simulink model "wetCondition scenario 3"  (R2025a)
settings: Solver=VariableStepAuto  StartTime=0.0  StopTime=10.0  RelTol=1e-3
libraries: SignalEditorBlockLib x5
settings Model: Creator=josik  LastModifiedBy=josik

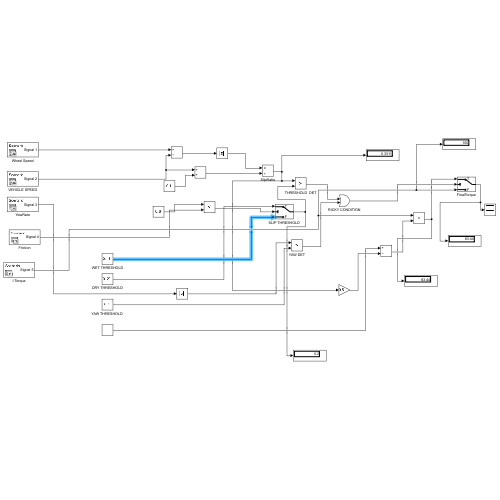
[thumbnail: Simulink's stored preview of the top-level diagram]
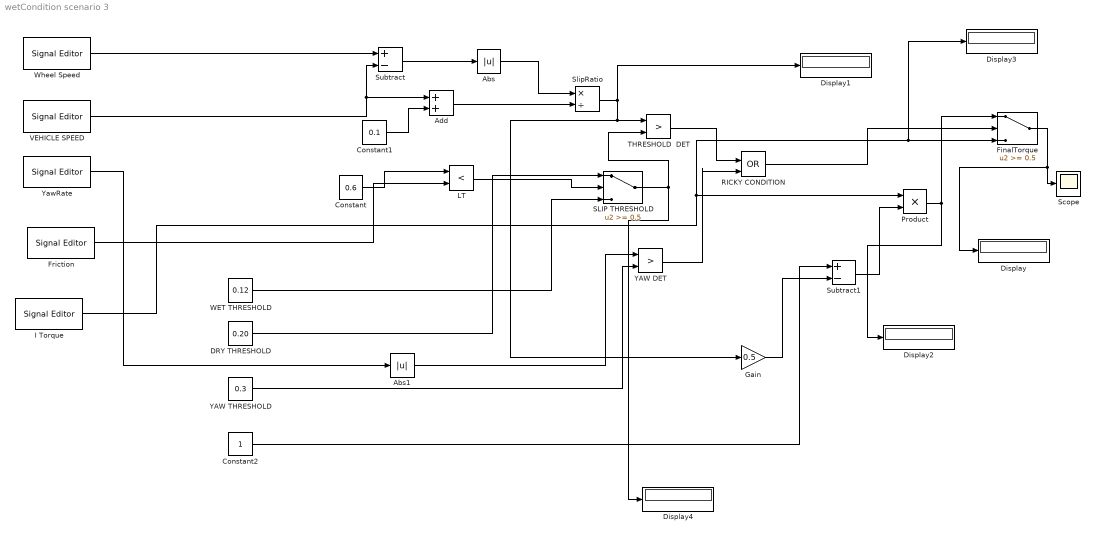
== system wetCondition scenario 3 ==
  Abs : Abs  SaturateOnIntegerOverflow=off
  Abs1 : Abs  SaturateOnIntegerOverflow=off
  Add : Sum
  Constant : Constant  Value=0.6
  Constant1 : Constant  Value=0.1
  Constant2 : Constant
  DRY THRESHOLD : Constant  Value=0.20
  Display{,1..4} (5 alike) : Display
  FinalTorque : Switch  Threshold=0.5  SaturateOnIntegerOverflow=off  InputSameDT=off
  Friction : SignalEditorBlockLib/Signal Editor  FileName=signal 4 sc 1.mat  ActiveScenario=Scenario  ActiveSignal=Signal 4  IsBus=off  OutputBusObjectStr=Bus: BusObject  SampleTime=0  ZeroCross=off  OutputAfterFinalValue=Setting to zero  Unit=inherit  PreserveSignalName=on  ApplySigPropsToAllScenarios=on  ApplySigPropsToAllSignals=off  SignalPropertySource=Dialog parameters
  Gain : Gain  Gain=0.5
  I Torque : SignalEditorBlockLib/Signal Editor  FileName=signal 5 sc 1.mat  ActiveScenario=Scenario  ActiveSignal=Signal 5  IsBus=off  OutputBusObjectStr=Bus: BusObject  SampleTime=0  ZeroCross=off  OutputAfterFinalValue=Setting to zero  Unit=inherit  PreserveSignalName=on  ApplySigPropsToAllScenarios=on  ApplySigPropsToAllSignals=off  SignalPropertySource=Dialog parameters
  LT : RelationalOperator  Operator=<  OutDataTypeStr=boolean  RndMeth=Simplest  InputSameDT=off
  Product : Product
  RICKY CONDITION : Logic  Operator=OR  IconShape=distinctive  AllPortsSameDT=off  OutDataTypeStr=boolean
  SLIP THRESHOLD : Switch  Threshold=0.5  SaturateOnIntegerOverflow=off  InputSameDT=off
  Scope : Scope
      settings: ActiveDisplayYMinimum=-50.978468435458396  ActiveDisplayYMaximum=144.98501047694566
  SlipRatio : Product  Inputs=*/
  Subtract : Sum  Inputs=+-
  Subtract1 : Sum  Inputs=+-
  THRESHOLD  DET : RelationalOperator  Operator=>  OutDataTypeStr=boolean  RndMeth=Simplest  InputSameDT=off
  VEHICLE SPEED : SignalEditorBlockLib/Signal Editor  FileName=signal 2 sc 1.mat  ActiveScenario=Scenario  ActiveSignal=Signal 2  IsBus=off  OutputBusObjectStr=Bus: BusObject  SampleTime=0  ZeroCross=off  OutputAfterFinalValue=Setting to zero  Unit=inherit  PreserveSignalName=on  ApplySigPropsToAllScenarios=on  ApplySigPropsToAllSignals=off  SignalPropertySource=Dialog parameters
  WET THRESHOLD : Constant  Value=0.12
  Wheel Speed : SignalEditorBlockLib/Signal Editor  FileName=signal 1 sc 1.mat  ActiveScenario=Scenario  ActiveSignal=Signal 1  IsBus=off  OutputBusObjectStr=Bus: BusObject  SampleTime=0  ZeroCross=off  OutputAfterFinalValue=Setting to zero  Unit=inherit  PreserveSignalName=on  ApplySigPropsToAllScenarios=on  ApplySigPropsToAllSignals=off  SignalPropertySource=Dialog parameters
  YAW DET : RelationalOperator  Operator=>  OutDataTypeStr=boolean  RndMeth=Simplest  InputSameDT=off
  "YAW THRESHOLD " : Constant  Value=0.3
  YawRate : SignalEditorBlockLib/Signal Editor  FileName=signal 3 sc 1.mat  ActiveScenario=Scenario  ActiveSignal=Signal 3  IsBus=off  OutputBusObjectStr=Bus: BusObject  SampleTime=0  ZeroCross=off  OutputAfterFinalValue=Setting to zero  Unit=inherit  PreserveSignalName=on  ApplySigPropsToAllScenarios=on  ApplySigPropsToAllSignals=off  SignalPropertySource=Dialog parameters
  wires:
  Wheel Speed/1 -> Subtract/1
  VEHICLE SPEED/1 -> Subtract/2, Add/1
  Subtract/1 -> Abs/1
  Constant1/1 -> Add/2
  Constant/1 -> LT/1
  WET THRESHOLD/1 -> SLIP THRESHOLD/3
  LT/1 -> SLIP THRESHOLD/2
  DRY THRESHOLD/1 -> SLIP THRESHOLD/1
  SlipRatio/1 -> THRESHOLD  DET/1, Gain/1, Display1/1
  YawRate/1 -> Abs1/1
  Abs1/1 -> YAW DET/1
  "YAW THRESHOLD "/1 -> YAW DET/2
  THRESHOLD  DET/1 -> RICKY CONDITION/1
  YAW DET/1 -> RICKY CONDITION/2
  Constant2/1 -> Subtract1/1
  Gain/1 -> Subtract1/2
  I Torque/1 -> Product/1, Display3/1, FinalTorque/3
  Subtract1/1 -> Product/2
  Product/1 -> Display2/1, FinalTorque/1
  RICKY CONDITION/1 -> FinalTorque/2
  SLIP THRESHOLD/1 -> THRESHOLD  DET/2, Display4/1
  Abs/1 -> SlipRatio/1
  Add/1 -> SlipRatio/2
  FinalTorque/1 -> Display/1, Scope/1
  Friction/1 -> LT/2
